simulink model "sprWid"  (R2016a)
settings: Solver=FixedStepDiscrete  StartTime=0.0  StopTime=inf  RelTol=1e-3
libraries: commdigbbndpm3 x2, commfilt2 x2, commrandsrc2 x1, commutil2 x1, commdigbbndam3 x1, dspsigops x1
settings Model: Creator=sikor  LastModifiedBy=sikor
settings DataIOCC: LimitDataPoints=on  SaveFormat=Array
settings DebuggingCC: SolverPrmCheckMsg=warning
settings HardwareCC: ProdBitPerPointer=32  ProdLargestAtomicFloat=None  ProdIntDivRoundTo=Undefined  ProdEndianess=Unspecified  ProdWordSize=32  ProdHWDeviceType=32-bit Generic
settings ModelReferenceCC: PropagateSignalLabelsOutOfModel=off
settings ConfigComp: CovModelRefEnable=Off  CovSFcnEnable=off

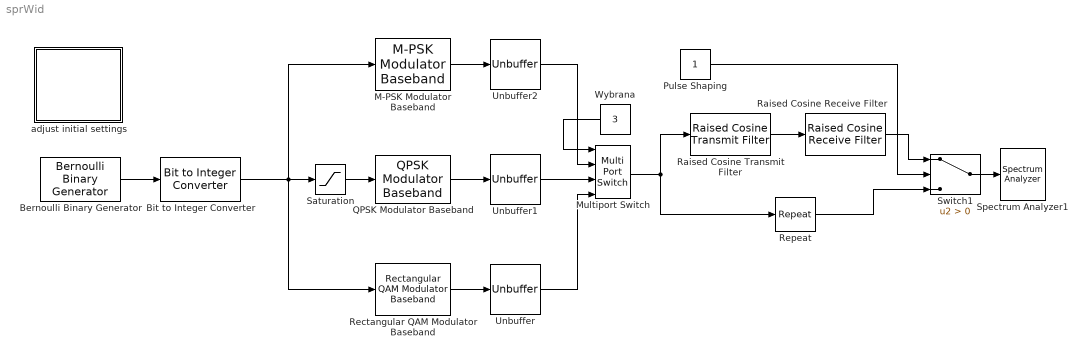
== system sprWid ==
  Bernoulli Binary Generator : commrandsrc2/Bernoulli Binary Generator  P=0.5  seed=61  Ts=1e-2  frameBased=on  sampPerFrame=6  orient=off  outDataType=boolean
  Bit to Integer Converter : commutil2/Bit to Integer Converter  nbits=6  bitOrder=MSB first  signedOutputValues=Unsigned  outDtype=int16  outDtypeSigned=Inherit via internal rule
  M-PSK Modulator Baseband : commdigbbndpm3/M-PSK Modulator Baseband  M=64  InType=Integer  Enc=Gray  Mapping=[0:7]  Ph=pi/8  outDtype=double  outWordLen=16  outUDDataType=sfix(16)  outFracLenMode=Best precision  outFracLen=15  outDataTypeStr=double  outLastDataTypeStr=double
  Multiport Switch : MultiPortSwitch  InputSameDT=on
  Pulse Shaping : Constant
  QPSK Modulator Baseband : commdigbbndpm3/QPSK Modulator Baseband  InType=Integer  Enc=Gray  Ph=pi/4  outDtype=double  outWordLen=16  outUDDataType=sfix(16)  outFracLenMode=Best precision  outFracLen=15  outDataTypeStr=double  outLastDataTypeStr=double
  Raised Cosine Receive Filter : commfilt2/Raised Cosine Receive Filter  filtType=Square root  R=0.15  filtSpan=10  N=16  downFactor=1  downOffset=0  filterGain=1  InputProcessing=Columns as channels (frame based)  RateOptions=Allow multirate processing  framing=Mute  checkCoeff=off  variableName=rcRxFilt  currentFiltSpan=10  D=5  inputOffset=0  sampMode=Mute  saveAsFlag=0  rateMode=Downsampling  checkGain=Normalized  launchFVT=on  roundingMode=Floor  overflowMode=off  coeffDataTypeStr=Inherit: Same word length as input  coeffMin=[]  coeffMax=[]  coeffLastDataTypeStr=Inherit: Same word length as input  accumDataTypeStr=Inherit: Same as product output  accumLastDataTypeStr=Inherit: Same as product output  outputDataTypeStr=Inherit: Same as accumulator  outputMin=[]  outputMax=[]  outputLastDataTypeStr=Inherit: Same as accumulator
  Raised Cosine Transmit Filter : commfilt2/Raised Cosine Transmit Filter  filtType=Square root  R=0.15  filtSpan=10  N=16  filterGain=1  InputProcessing=Columns as channels (frame based)  RateOptions=Allow multirate processing  framing=Mute  checkCoeff=off  variableName=rcTxFilt1  checkGain=Normalized  sampMode=Mute  saveAsFlag=0  currentFiltSpan=10  D=(10)/2  launchFVT=on  roundingMode=Floor  overflowMode=off  coeffDataTypeStr=Inherit: Same word length as input  coeffMin=[]  coeffMax=[]  coeffLastDataTypeStr=Inherit: Same word length as input  outputDataTypeStr=Inherit: Same as accumulator  outputMin=[]  outputMax=[]  outputLastDataTypeStr=Inherit: Same as accumulator
  Rectangular QAM Modulator Baseband : commdigbbndam3/Rectangular QAM Modulator Baseband  M=64  InType=Integer  Enc=Gray  Mapping=[0:15]  PowType=Min. distance between symbols  MinDist=2  AvgPow=1  PeakPow=1  Ph=0  outDtype=double  outWordLen=16  outUDDataType=sfix(16)  outFracLenMode=Best precision  outFracLen=15  outDataTypeStr=double  outLastDataTypeStr=double
  Repeat : dspsigops/Repeat  N=16  InputProcessing=Columns as channels (frame based)  RateOptions=Allow multirate processing  ic=0  mode=Unused parameter value
  Saturation : Saturate  UpperLimit=3  LowerLimit=0
  Spectrum Analyzer1 : SpectrumAnalyzer
  Switch1 : Switch  Criteria=u2 > Threshold
  Unbuffer : Unbuffer  SampleBasedProcessing=Same as frame based
  Unbuffer1 : Unbuffer  SampleBasedProcessing=Same as frame based
  Unbuffer2 : Unbuffer  SampleBasedProcessing=Same as frame based
  Wybrana : Constant  Value=3
  adjust initial settings : Subsystem  mask(RF Link Demo:Initial Settings){modType=64 QAM, rcEnabled=on, rolloffFactor=0.15}
      mask prompts: modType "Modulation type:"; rcEnabled "Pulse Shaping"; rolloffFactor "0.35"
      mask help: Select the scenarios from the mask to change the link parameters. Each of the mask parameters sets the parameters in the corresponding RF impairment block(s).
      mask init:
      | if rcEnabled
      |          set_param('sprWid/Pulse Shaping','Value','1')
      |     else
      |          set_param('sprWid/Pulse Shaping','Value','0')        
      |     end
      | 
      | 
      | if rolloffFactor <=0
      |     rolloffFactor=0.1;
      | end
      | 
      | if rolloffFactor >=1.0
      |     rolloffFactor=0.99;
      | end
      | 
      | set_param('sprWid/Raised Cosine Receive Filter','R',sprintf('%g',rolloffFactor))
      | set_param('sprWid/Raised Cosine Transmit Filter','R',sprintf('%g',rolloffFactor))
      | 
      | 
      | 
      |     switch modType
      |         case 1, %64 PSK
      |          set_param('sprWid/Bernoulli Binary Generator','sampPerFrame','6')
      |          set_param('sprWid/Bit to Integer Converter','nbits','6')
      |          set_param('sprWid/Wybrana','Value','1')
      |         case 2, %QPSK
      |          set_param('sprWid/Bernoulli Binary Generator','sampPerFrame','2')
      |          set_param('sprWid/Bit to Integer Converter','nbits','2')
      |          set_param('sprWid/Wybrana','Value','2')         
      |         case 3, %64 QAM
      |          set_param('sprWid/Bernoulli Binary Generator','sampPerFrame','6')
      |          set_param('sprWid/Bit to Integer Converter','nbits','6')
      |          set_param('sprWid/Wybrana','Value','3')         
      |     end
      mask TypeOptions modType: 64 PSK | QPSK | 64 QAM
      mask Display: disp('Spectral Efficiency');
  wires:
  Bernoulli Binary Generator/1 -> Bit to Integer Converter/1
  M-PSK Modulator Baseband/1 -> Unbuffer2/1
  Bit to Integer Converter/1 -> Rectangular QAM Modulator Baseband/1, Saturation/1, M-PSK Modulator Baseband/1
  QPSK Modulator Baseband/1 -> Unbuffer1/1
  Rectangular QAM Modulator Baseband/1 -> Unbuffer/1
  Unbuffer/1 -> Multiport Switch/4
  Unbuffer1/1 -> Multiport Switch/3
  Unbuffer2/1 -> Multiport Switch/2
  Wybrana/1 -> Multiport Switch/1
  Saturation/1 -> QPSK Modulator Baseband/1
  Raised Cosine Transmit Filter/1 -> Raised Cosine Receive Filter/1
  Switch1/1 -> Spectrum Analyzer1/1
  Raised Cosine Receive Filter/1 -> Switch1/1
  Repeat/1 -> Switch1/3
  Multiport Switch/1 -> Repeat/1, Raised Cosine Transmit Filter/1
  Pulse Shaping/1 -> Switch1/2

== system sprWid/adjust initial settings ==
